simulink model "BoundedTorqueControl"  (Simulink 8.6)
settings: Solver=FixedStepDiscrete  StartTime=0.0  StopTime=CONFIG.SIMULATION_TIME  FixedStep=CONFIG.Ts  RelTol=1e-3
InitFcn:
  | cd(fileparts(which(bdroot)));
  | init_BoundedTorqueControl;
StopFcn:
  | visualization
values from neighbouring files (symbols this model uses):
  q0 = zeros(model.n, 1)    [gains.m]
  qd0 = zeros(model.n, 1)    [gains.m]
  ROBOT_DOF = model.n    [gains.m]
  ROBOT_DOF_SIM = eye(ROBOT_DOF)    [gains.m]
undefined symbols (not defined in the file or in its folder): CONFIG, DiscIntNeverNeededParam, model
settings Model: Creator=marie  LastModifiedBy=marie
settings DataIOCC: SaveFormat=StructureWithTime  SignalLoggingSaveFormat=Dataset
settings OptimizationCC: ExpressionDepthLimit=128
settings DebuggingCC: UnderspecifiedInitializationDetection=Simplified  MergeDetectMultiDrivingBlocksExec=error  SolverPrmCheckMsg=none  FcnCallInpInsideContextMsg=EnableAllAsError  StateNameClashWarn=none
settings HardwareCC: ProdBitPerPointer=64  ProdLargestAtomicFloat=Float  ProdIntDivRoundTo=Zero  ProdEndianess=LittleEndian  ProdHWDeviceType=Specified
settings GRTTargetCC: GeneratePreprocessorConditionals=Use local settings  CombineOutputUpdateFcns=on  GRTInterface=off
settings ConfigComp: CovModelRefEnable=off

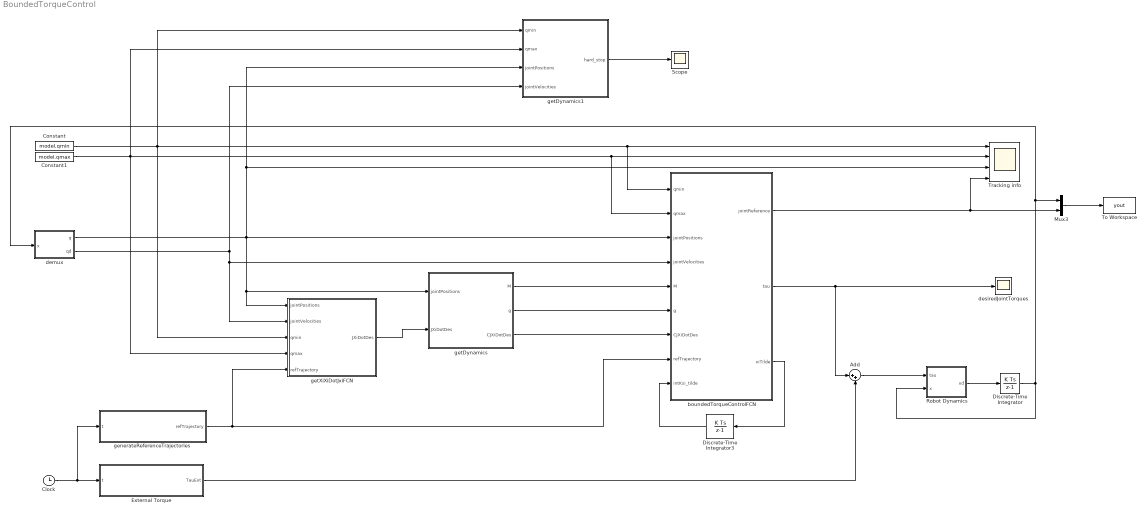
== system BoundedTorqueControl ==
  Add : Sum  Inputs=|++
  Clock : Clock
  Constant : Constant  Value=model.qmin
  Constant1 : Constant  Value=model.qmax
  Discrete-Time Integrator : DiscreteIntegrator  InitialCondition=[q0; qd0]  SampleTime=CONFIG.Ts  ICPrevOutput=DiscIntNeverNeededParam  ICPrevScaledInput=DiscIntNeverNeededParam
  Discrete-Time Integrator3 : DiscreteIntegrator  InitialCondition=zeros(ROBOT_DOF,1)  SampleTime=CONFIG.Ts  ICPrevOutput=DiscIntNeverNeededParam  ICPrevScaledInput=DiscIntNeverNeededParam
  External Torque : MATLAB Function  TreatAsAtomicUnit=on
  Mux3 : Mux  Inputs=2
  Robot Dynamics : MATLAB Function  TreatAsAtomicUnit=on
  Scope : Scope
  To Workspace : ToWorkspace  VariableName=yout  SaveFormat=Structure With Time  SampleTime=-1
  Tracking info : Scope  NumInputPorts=4
  boundedTorqueControlFCN : MATLAB Function  TreatAsAtomicUnit=on
  demux : MATLAB Function  TreatAsAtomicUnit=on
  desiredJointTorques : Scope
  generateReferenceTrajectories : MATLAB Function  TreatAsAtomicUnit=on
  getDynamics : MATLAB Function  TreatAsAtomicUnit=on
  getDynamics1 : MATLAB Function  TreatAsAtomicUnit=on
  getXiXiDotJxiFCN : MATLAB Function  TreatAsAtomicUnit=on
  wires:
  demux/1(q) -> getDynamics/1(jointPositions), getXiXiDotJxiFCN/1(jointPositions), boundedTorqueControlFCN/3(jointPositions), getDynamics1/3(jointPositions), Tracking info/3
  demux/2(qd) -> getDynamics1/4(jointVelocities), boundedTorqueControlFCN/4(jointVelocities), getXiXiDotJxiFCN/2(jointVelocities)
  getDynamics/1(M) -> boundedTorqueControlFCN/5(M)
  Constant1/1 -> getDynamics1/2(qmax), getXiXiDotJxiFCN/4(qmax), boundedTorqueControlFCN/2(qmax), Tracking info/2
  Constant/1 -> getDynamics1/1(qmin), boundedTorqueControlFCN/1(qmin), Tracking info/1, getXiXiDotJxiFCN/3(qmin)
  boundedTorqueControlFCN/2(tau) -> Add/1, desiredJointTorques/1
  Discrete-Time Integrator3/1 -> boundedTorqueControlFCN/9(intKsi_tilde)
  Clock/1 -> generateReferenceTrajectories/1(t), External Torque/1(t)
  External Torque/1(TauExt) -> Add/2
  boundedTorqueControlFCN/1(jointReference) -> Tracking info/4, Mux3/2
  getDynamics/2(g) -> boundedTorqueControlFCN/6(g)
  getXiXiDotJxiFCN/1(JXiDotDes) -> getDynamics/2(JXiDotDes)
  getDynamics/3(CJXiDotDes) -> boundedTorqueControlFCN/7(CJXiDotDes)
  boundedTorqueControlFCN/3(xiTilde) -> Discrete-Time Integrator3/1
  Add/1 -> Robot Dynamics/1(tau)
  Robot Dynamics/1(xd) -> Discrete-Time Integrator/1
  Discrete-Time Integrator/1 -> demux/1(x), Mux3/1, Robot Dynamics/2(x)
  Mux3/1 -> To Workspace/1
  generateReferenceTrajectories/1(refTrajectory) -> getXiXiDotJxiFCN/5(refTrajectory), boundedTorqueControlFCN/8(refTrajectory)
  getDynamics1/1(hard_stop) -> Scope/1

== matlab function boundedTorqueControlFCN ==
  data: model parameter double; qmin input double; qmax input double; jointReference output double; jointPositions input double; jointVelocities input double; M input double; g input double; CJXiDotDes input double; refTrajectory input double; intKsi_tilde input double; tau output double; xiTilde output double
function [jointReference, tau, xiTilde] =  boundedJointEvolutionControl(model, qmin, qmax, jointPositions, jointVelocities, M, g, CJXiDotDes, refTrajectory, intKsi_tilde)


    [~, ~, jointReference, ~, tau, xiTilde] = boundedJointEvolutionControl(model, qmin, qmax, jointPositions, jointVelocities, M, g, CJXiDotDes, refTrajectory, intKsi_tilde);

== matlab function generateReferenceTrajectories ==
  data: refTrajectory output double; t input double; model parameter double; ROBOT_DOF_SIM parameter double
function refTrajectory  = generateReferenceTrajectoriesFCN(t, model,ROBOT_DOF_SIM)

% refTrajectory  = ones(size(ROBOT_DOF_SIM,1),1)*generateReferenceTrajectories(t, model);

refTrajectory  = generateReferenceTrajectories(t, model);

== matlab function External Torque ==
  data: TauExt output double; t input double; model parameter double
function TauExt = applyExternTorqueFCN(t, model)

TauExt = applyExternTorque(t, model);

== matlab function getXiXiDotJxiFCN ==
  data: JXiDotDes output double; jointPositions input double; jointVelocities input double; qmin input double; qmax input double; refTrajectory input double
function JXiDotDes  = getXiXiDotJxiFCN(jointPositions,jointVelocities, qmin, qmax, refTrajectory)


[~,~,J,~]        = getXiXiDotJxi(jointPositions,jointVelocities,qmin, qmax);

[r,rDot,~]       = getReferences(refTrajectory);

[~,xiDotDes,~,~] = getXiXiDotJxi(r,rDot,qmin, qmax);

JXiDotDes        = J*xiDotDes;

== matlab function Robot Dynamics ==
  data: tau input double; x input double; xd output double; model parameter double
function xd = getDyn(tau, x, model)

%Compute the dynamics of the system, 
%from the parameters in model
%following Siciliano, p.268

%Input:
%Tau: control torques
%x = [q; qd] = [x1; x2]
%model: model parameters set in init script

%Output:
%xd = [qd; qdd] = [x2; M\(tau - h(q,qd))]

q = x(1:2);
qd = x(3:4);

Fv = model.Fv;

%M matrix
M = computeMSiciliano(q,model);

%C matrix
C = computeCSiciliano(q,qd,model);

%G matrix
G = computeGSiciliano(q, model);


qdd = M \ (tau - C*qd - Fv*qd - G);

xd = [qd; qdd];

end

== matlab function getDynamics ==
  data: jointPositions input double; JXiDotDes input double; M output double; g output double; CJXiDotDes output double; model parameter double
function [M, g, CJXiDotDes] = getDynamics(jointPositions, JXiDotDes, model)


M = computeMSiciliano(jointPositions, model);

g = computeGSiciliano(jointPositions, model);

CJXiDotDes = computeCSiciliano(jointPositions, JXiDotDes, model) * JXiDotDes;

== matlab function demux ==
  data: x input double; q output double; qd output double
function [q, qd] = getq(x)

%From the dynamics output x, extract the joint positions and velocities

%Input
%x: state of the system in the form [q;qd], output from the dynamic model

%Output
%q: joint positions
%qd: joint velocities

q = x(1:2);
q(1) = q(1);
qd = x(3:4);

== matlab function getDynamics1 ==
  data: qmin input double; qmax input double; jointPositions input double; hard_stop output double; jointVelocities input double; ROBOT_DOF parameter double
function hard_stop = getDynamics(qmin, qmax, jointPositions, jointVelocities, ROBOT_DOF)

hard_stop = zeros(ROBOT_DOF, 1);

%Coefficients
a = 1e4;
b = 1;

for i = 1 : ROBOT_DOF
   
    if jointPositions(i) <= qmin(i)
%         y = jointPositions(i) - qmin(i);
        hard_stop(i) = a * (abs(jointPositions(i) - qmin(i)))^3 * (1 - b * jointVelocities(i));
    elseif jointPositions(i) >= qmax(i)
%         y = qmax(i) - jointPositions(i);
        hard_stop(i) = a * (abs(qmax(i) - jointPositions(i)))^3 * (1 - b * jointVelocities(i));
    else
        hard_stop(i) = 0;
    end
    
end
